simulink model "MPCRLTestPredict"  (R2023a)
settings: Solver=ode1  StartTime=0.0  StopTime=10  FixedStep=0.005  RelTol=1e-3  EnableMultiTasking=on
values from neighbouring files (symbols this model uses):
  bp = 5e-5*2    (= 0.0001)    [Copy_of_qube2_rotpen_param.m]    (also in MPCmodelinitial.m = 5e-05)
  br = 1e-3*2    (= 0.002)    [Copy_of_qube2_rotpen_param.m]    (also in MPCmodelinitial.m = 0.001)
  g = 9.81    [Copy_of_qube2_rotpen_param.m]    (also in MPCmodelinitial.m)
  Jp = mp*Lp^2/3    (= 0.0001464408)    [Copy_of_qube2_rotpen_param.m]    (also in MPCmodelinitial.m = 0.000133128)
  Jr = mr*r^2/3    (= 0.000251670833333)    [Copy_of_qube2_rotpen_param.m]    (also in MPCmodelinitial.m = 0.000228791666667)
  km = kt    (= 0.042)    [Copy_of_qube2_rotpen_param.m]    (also in MPCmodelinitial.m)
  kt = 0.042    [Copy_of_qube2_rotpen_param.m]    (also in MPCmodelinitial.m)
  l = Lp/2    (= 0.0645)    [Copy_of_qube2_rotpen_param.m]    (also in MPCmodelinitial.m)
  mp = 0.024*1.1    (= 0.0264)    [Copy_of_qube2_rotpen_param.m]    (also in MPCmodelinitial.m = 0.024)
  r = 0.085    [Copy_of_qube2_rotpen_param.m]    (also in MPCmodelinitial.m)
  Rm = 9.7    [Copy_of_qube2_rotpen_param.m]    (also in MPCmodelinitial.m = 8.4)
undefined symbols (not defined in the file or in its folder): ic_alpha0
libraries: simulink x6, rllib x3, sdolib x3, mpclib x2
settings Model: PacingRate=1000  ExtModeTrigDuration=10000  Creator=XIJ62  LastModifiedBy=lying
settings SolverCC: AlgebraicLoopSolver=TrustRegion  PositivePriorityOrder=on
settings DataIOCC: ReturnWorkspaceOutputs=off
settings DebuggingCC: UnconnectedInputMsg=warning  UnconnectedOutputMsg=warning  UnconnectedLineMsg=warning  ArithmeticOperatorsInVariantConditions=warning
settings ModelReferenceCC: EnableRefExpFcnMdlSchedulingChecks=on
settings SFSimCC: SimUseLocalCustomCode=off  CustomCodeUndefinedFunction=UseInterfaceOnly
settings RTWCC: Description=QUARC Win64 Target Using Toolchain  SystemTargetFile=quarc_win64.tlc  TemplateMakefile=quarc_default_tmf  RTWUseLocalCustomCode=off  Toolchain=QUARC win64 | nmake (64-bit Windows)  BuildConfiguration=Faster Runs  DLArmComputeVersion=19.05
settings CodeAppCC: StateflowObjectComments=on
settings STFCustomTargetCC: SystemTargetFile=quarc_win64.tlc
settings GRTTargetCC: ParMdlRefBuildCompliant=off  CompOptLevelCompliant=off  CombineOutputUpdateFcns=off  MatFileLogging=off  CPPClassGenCompliant=off  GRTInterface=on  ExtMode=on  ExtModeMexFile=quarc_comm
settings ConfigComp: CovMetricSettings=dswe

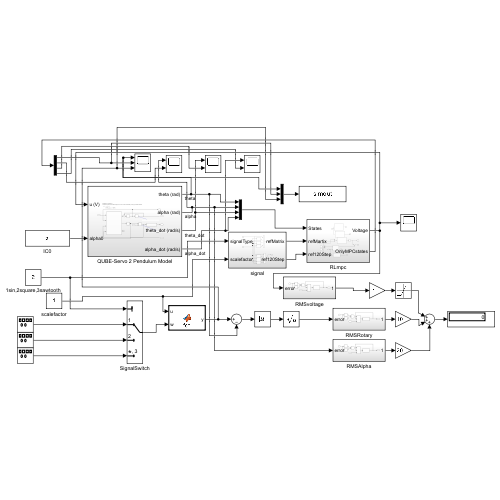
[thumbnail: Simulink's stored preview of the top-level diagram]
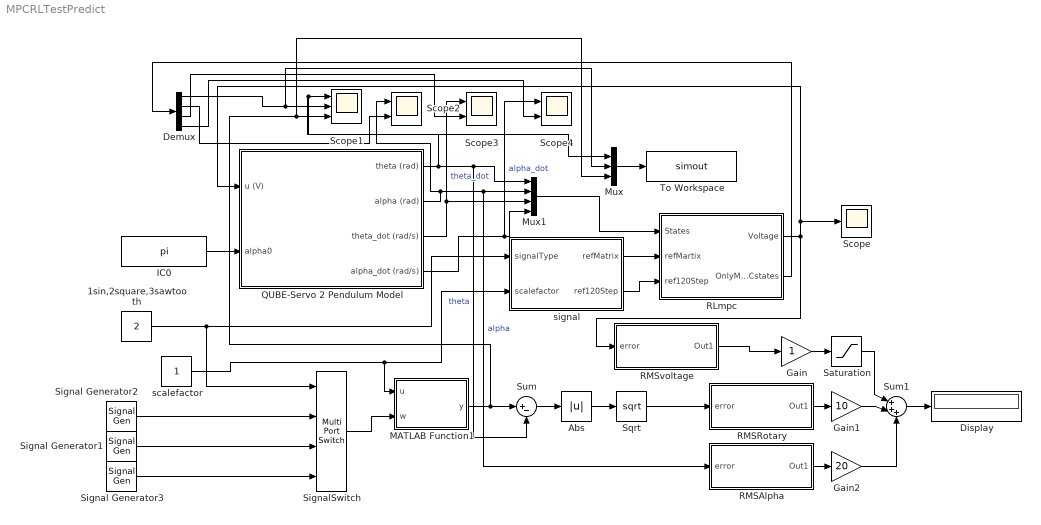
== system MPCRLTestPredict ==
  1sin,2square,3sawtooth : Constant  Value=2
  Abs : Abs  SaturateOnIntegerOverflow=off
  Demux : Demux
  Display : Display
  Gain : Gain
  Gain1 : Gain  Gain=10
  Gain2 : Gain  Gain=20
  IC0 : Constant  Value=pi
  MATLAB Function1 : MATLAB Function  TreatAsAtomicUnit=on
  Mux : Mux  Inputs=3
  Mux1 : Mux
  QUBE-Servo 2 Pendulum Model : Subsystem
  RLmpc : Subsystem
  RMSAlpha : Subsystem
  RMSRotary : Subsystem
  RMSvoltage : Subsystem
  Saturation : Saturate  UpperLimit=0  LowerLimit=0
  Scope : Scope
  Scope1 : Scope  NumInputPorts=3
  Scope2 : Scope  NumInputPorts=2
  Scope3 : Scope  NumInputPorts=2
  Scope4 : Scope  NumInputPorts=2
  Signal Generator1 : SignalGenerator  WaveForm=square  Amplitude=0.5  Units=rad/sec
  Signal Generator2 : SignalGenerator  Units=rad/sec
  Signal Generator3 : SignalGenerator  WaveForm=sawtooth  Units=rad/sec
  SignalSwitch : MultiPortSwitch  SaturateOnIntegerOverflow=off  InputSameDT=off
  Sqrt : Sqrt
  Sum : Sum  Inputs=|+-
  Sum1 : Sum  Inputs=|+++
  To Workspace : ToWorkspace  VariableName=simout  SaveFormat=Timeseries  SampleTime=-1
  scalefactor : Constant
  signal : Subsystem
  wires:
  RLmpc/1(Voltage) -> QUBE-Servo 2 Pendulum Model/1(u (V)), Scope/1, RMSvoltage/1(error)
  QUBE-Servo 2 Pendulum Model/1(theta (rad)) -> Mux/1, Scope1/1, Mux1/1, Sum/2  "theta"
  QUBE-Servo 2 Pendulum Model/2(alpha (rad)) -> Scope2/1, RMSAlpha/1(error), Mux1/2  "alpha"
  QUBE-Servo 2 Pendulum Model/3(theta_dot (rad/s)) -> Scope3/1, Mux1/3  "theta_dot"
  QUBE-Servo 2 Pendulum Model/4(alpha_dot (rad/s)) -> Scope4/1, Mux1/4  "alpha_dot"
  Mux1/1 -> RLmpc/1(States)
  IC0/1 -> QUBE-Servo 2 Pendulum Model/2(alpha0)
  RMSRotary/1(Out1) -> Gain1/1
  Sum/1 -> Abs/1
  scalefactor/1 -> MATLAB Function1/1(u), signal/2(scalefactor)
  signal/1(refMatrix) -> RLmpc/2(refMartix)
  signal/2(ref120Step) -> RLmpc/3(ref120Step)
  SignalSwitch/1 -> MATLAB Function1/2(w)
  MATLAB Function1/1(y) -> Sum/1, Mux/3, Scope1/3
  Signal Generator1/1 -> SignalSwitch/3
  Signal Generator2/1 -> SignalSwitch/2
  1sin,2square,3sawtooth/1 -> SignalSwitch/1, signal/1(signalType)
  RMSvoltage/1(Out1) -> Gain/1
  Signal Generator3/1 -> SignalSwitch/4
  RLmpc/2(OnlyMPCstates) -> Demux/1
  Demux/1 -> Mux/2, Scope1/2
  Demux/2 -> Scope2/2
  Demux/3 -> Scope3/2
  Demux/4 -> Scope4/2
  Mux/1 -> To Workspace/1
  RMSAlpha/1(Out1) -> Gain2/1
  Gain/1 -> Saturation/1
  Gain1/1 -> Sum1/2
  Gain2/1 -> Sum1/3
  Sum1/1 -> Display/1
  Abs/1 -> Sqrt/1
  Sqrt/1 -> RMSRotary/1(error)
  Saturation/1 -> Sum1/1

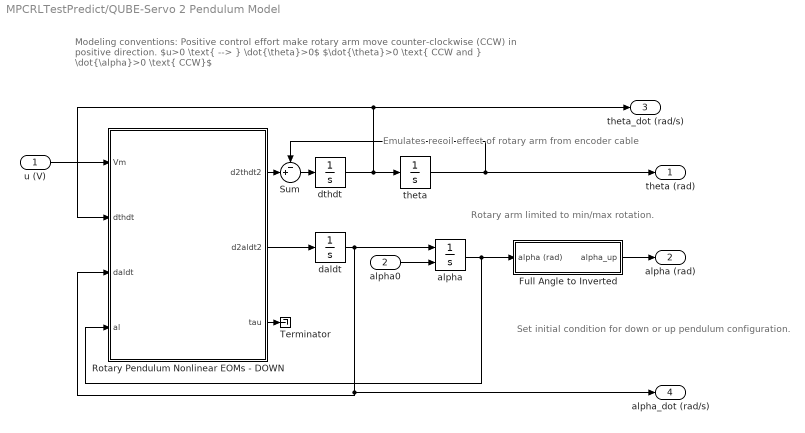
== system MPCRLTestPredict/QUBE-Servo 2 Pendulum Model ==
  note: Rotary arm limited to min/max rotation.
  note: Modeling conventions:
      | Positive control effort make rotary arm move counter-clockwise (CCW) in positive direction.
      | $u>0 \text{ --> } \dot{\theta}>0$
      | $\dot{\theta}>0 \text{ CCW and } \dot{\alpha}>0 \text{ CCW}$
  note: Set initial condition for down or up pendulum configuration.
  note: Emulates recoil effect of rotary arm from encoder cable
  u (V) : Inport
  alpha0 : Inport  Port=2
  Full Angle to Inverted : Subsystem
  Rotary Pendulum Nonlinear EOMs - DOWN : MATLAB Function  TreatAsAtomicUnit=on
  Sum : Sum  Inputs=-+|
  Terminator : Terminator
  alpha : Integrator  InitialConditionSource=external  InitialCondition=ic_alpha0
  daldt : Integrator
  dthdt : Integrator
  theta : Integrator  LimitOutput=on  UpperSaturationLimit=2  LowerSaturationLimit=-2
  theta (rad) : Outport  VectorParamsAs1DForOutWhenUnconnected=off
  alpha (rad) : Outport  Port=2  VectorParamsAs1DForOutWhenUnconnected=off
  theta_dot (rad/s) : Outport  Port=3  VectorParamsAs1DForOutWhenUnconnected=off
  alpha_dot (rad/s) : Outport  Port=4  VectorParamsAs1DForOutWhenUnconnected=off
  wires:
  daldt/1 -> Rotary Pendulum Nonlinear EOMs - DOWN/3(daldt), alpha_dot (rad/s)/1, alpha/1
  alpha/1 -> Full Angle to Inverted/1(alpha (rad)), Rotary Pendulum Nonlinear EOMs - DOWN/4(al)
  Rotary Pendulum Nonlinear EOMs - DOWN/2(d2aldt2) -> daldt/1
  dthdt/1 -> theta_dot (rad/s)/1, Rotary Pendulum Nonlinear EOMs - DOWN/2(dthdt), theta/1
  u (V)/1 -> Rotary Pendulum Nonlinear EOMs - DOWN/1(Vm)
  Rotary Pendulum Nonlinear EOMs - DOWN/3(tau) -> Terminator/1
  Full Angle to Inverted/1(alpha_up) -> alpha (rad)/1
  alpha0/1 -> alpha/2
  theta/1 -> theta (rad)/1, Sum/1
  Rotary Pendulum Nonlinear EOMs - DOWN/1(d2thdt2) -> Sum/2
  Sum/1 -> dthdt/1

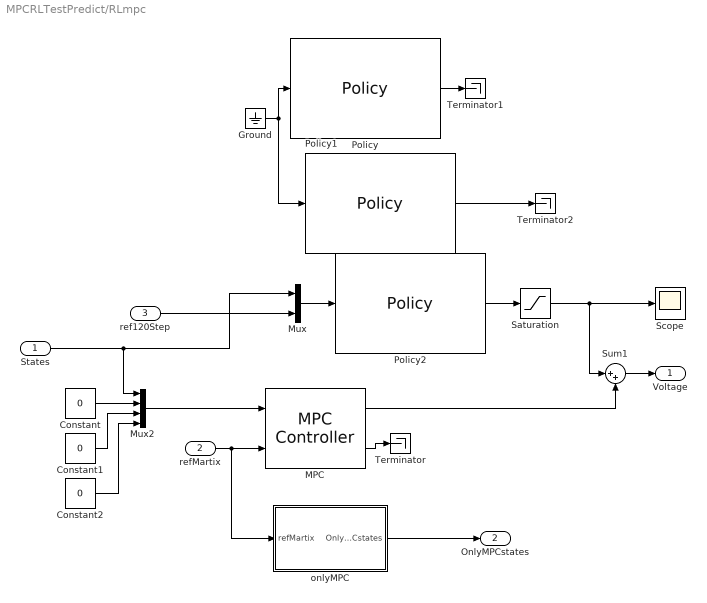
== system MPCRLTestPredict/RLmpc ==
  States : Inport
  refMartix : Inport  Port=2
  ref120Step : Inport  Port=3
  Constant : Constant  Value=0
  Constant1 : Constant  Value=0
  Constant2 : Constant  Value=0
  Ground : Ground
  MPC : mpclib/MPC Controller  SCDEnableBlockLinearizationSpecification=on  mpcobj=mpc1  is_multiple=0  enable_value=0  return_u0=off  updateMPCinCallerWorkspace=on  md_inport=off  mv_inport=off  uref_inport=off  return_cost=off  return_mvseq=off  return_qpstatus=off  return_xseq=off  return_state=on  return_ovseq=off  state_inport=on  umin_inport=off  umax_inport=off  ymin_inport=off  ymax_inport=off  cc_inport=off  ywt_inport=off  uwt_inport=off  duwt_inport=off  rhoeps_inport=off  pm_inport=off  MaximumP=10  HorizonChoice=FixedHorizon  n_ts=0.005  n_p=120  n_mv=1  n_md=0  n_ud=0  n_mo=4  n_uo=0  BlockDataType=double  SampleTimeInherited=off  switch_inport=off
  Mux : Mux  Inputs=2
  Mux2 : Mux
  Policy : rllib/Policy  MATFile=blockAgentData1.mat  SimUsingCodegen=off
  Policy1 : rllib/Policy  MATFile=blockAgentData2.mat  SimUsingCodegen=off
  Policy2 : rllib/Policy  MATFile=blockAgentData6.mat  SimUsingCodegen=off
  Saturation : Saturate  UpperLimit=10  LowerLimit=-10
  Scope : Scope
  Sum1 : Sum  Inputs=|++
  Terminator : Terminator
  Terminator1 : Terminator
  Terminator2 : Terminator
  onlyMPC : Subsystem
  Voltage : Outport
  OnlyMPCstates : Outport  Port=2
  wires:
  States/1 -> Mux2/1, Mux/1
  refMartix/1 -> onlyMPC/1(refMartix), MPC/2
  ref120Step/1 -> Mux/2
  MPC/2 -> Terminator/1
  MPC/1 -> Sum1/2
  Sum1/1 -> Voltage/1
  Constant1/1 -> Mux2/3
  Constant2/1 -> Mux2/4
  Constant/1 -> Mux2/2
  Mux2/1 -> MPC/1
  Saturation/1 -> Scope/1, Sum1/1
  onlyMPC/1(OnlyMPCstates) -> OnlyMPCstates/1
  Ground/1 -> Policy/1, Policy1/1
  Policy/1 -> Terminator1/1
  Policy1/1 -> Terminator2/1
  Mux/1 -> Policy2/1
  Policy2/1 -> Saturation/1

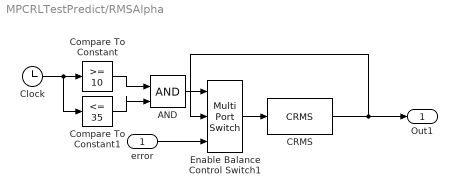
== system MPCRLTestPredict/RMSAlpha ==
  error : Inport
  AND : Logic  IconShape=distinctive  AllPortsSameDT=off  OutDataTypeStr=boolean
  CRMS : sdolib/RMS Blocks/CRMS
  Clock : Clock
  Compare To Constant : simulink/Logic and Bit Operations/Compare To Constant  relop=>=  const=10  OutDataTypeStr=boolean
  Compare To Constant1 : simulink/Logic and Bit Operations/Compare To Constant  relop=<=  const=35  OutDataTypeStr=boolean
  Enable Balance Control Switch1 : MultiPortSwitch  DataPortOrder=Zero-based contiguous  Inputs=2  zeroidx=on  SaturateOnIntegerOverflow=off  InputSameDT=off
  Out1 : Outport
  wires:
  Clock/1 -> Compare To Constant/1, Compare To Constant1/1
  Compare To Constant1/1 -> AND/2
  Compare To Constant/1 -> AND/1
  AND/1 -> Enable Balance Control Switch1/1
  Enable Balance Control Switch1/1 -> CRMS/1
  CRMS/1 -> Enable Balance Control Switch1/2, Out1/1
  error/1 -> Enable Balance Control Switch1/3

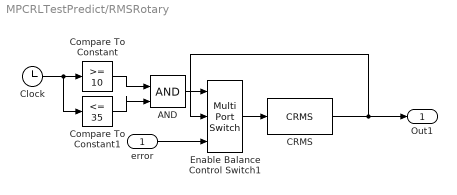
== system MPCRLTestPredict/RMSRotary ==
  error : Inport
  AND : Logic  IconShape=distinctive  AllPortsSameDT=off  OutDataTypeStr=boolean
  CRMS : sdolib/RMS Blocks/CRMS
  Clock : Clock
  Compare To Constant : simulink/Logic and Bit Operations/Compare To Constant  relop=>=  const=10  OutDataTypeStr=boolean
  Compare To Constant1 : simulink/Logic and Bit Operations/Compare To Constant  relop=<=  const=35  OutDataTypeStr=boolean
  Enable Balance Control Switch1 : MultiPortSwitch  DataPortOrder=Zero-based contiguous  Inputs=2  zeroidx=on  SaturateOnIntegerOverflow=off  InputSameDT=off
  Out1 : Outport
  wires:
  Clock/1 -> Compare To Constant/1, Compare To Constant1/1
  Compare To Constant1/1 -> AND/2
  Compare To Constant/1 -> AND/1
  AND/1 -> Enable Balance Control Switch1/1
  Enable Balance Control Switch1/1 -> CRMS/1
  CRMS/1 -> Enable Balance Control Switch1/2, Out1/1
  error/1 -> Enable Balance Control Switch1/3

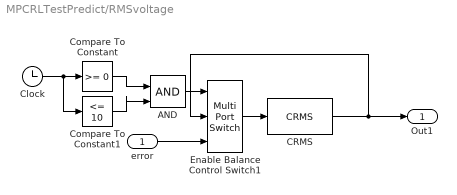
== system MPCRLTestPredict/RMSvoltage ==
  error : Inport
  AND : Logic  IconShape=distinctive  AllPortsSameDT=off  OutDataTypeStr=boolean
  CRMS : sdolib/RMS Blocks/CRMS
  Clock : Clock
  Compare To Constant : simulink/Logic and Bit Operations/Compare To Constant  relop=>=  const=0  OutDataTypeStr=boolean
  Compare To Constant1 : simulink/Logic and Bit Operations/Compare To Constant  relop=<=  const=10  OutDataTypeStr=boolean
  Enable Balance Control Switch1 : MultiPortSwitch  DataPortOrder=Zero-based contiguous  Inputs=2  zeroidx=on  SaturateOnIntegerOverflow=off  InputSameDT=off
  Out1 : Outport
  wires:
  Clock/1 -> Compare To Constant/1, Compare To Constant1/1
  Compare To Constant1/1 -> AND/2
  Compare To Constant/1 -> AND/1
  AND/1 -> Enable Balance Control Switch1/1
  Enable Balance Control Switch1/1 -> CRMS/1
  CRMS/1 -> Enable Balance Control Switch1/2, Out1/1
  error/1 -> Enable Balance Control Switch1/3

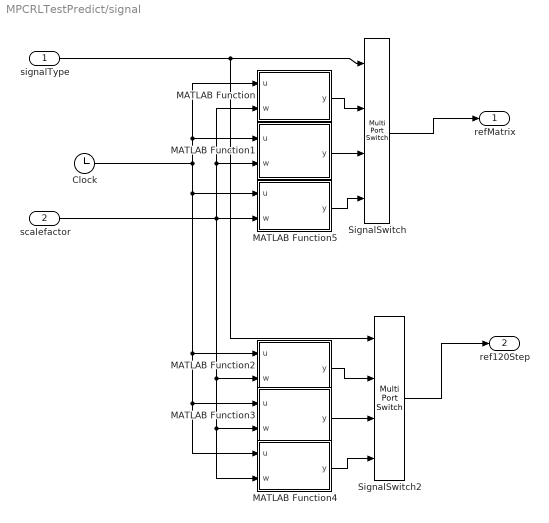
== system MPCRLTestPredict/signal ==
  signalType : Inport
  scalefactor : Inport  Port=2
  Clock : Clock
  MATLAB Function : MATLAB Function  TreatAsAtomicUnit=on
  MATLAB Function1 : MATLAB Function  TreatAsAtomicUnit=on
  MATLAB Function2 : MATLAB Function  TreatAsAtomicUnit=on
  MATLAB Function3 : MATLAB Function  TreatAsAtomicUnit=on
  MATLAB Function4 : MATLAB Function  TreatAsAtomicUnit=on
  MATLAB Function5 : MATLAB Function  TreatAsAtomicUnit=on
  SignalSwitch : MultiPortSwitch  SaturateOnIntegerOverflow=off  InputSameDT=off
  SignalSwitch2 : MultiPortSwitch  SaturateOnIntegerOverflow=off  InputSameDT=off
  refMatrix : Outport
  ref120Step : Outport  Port=2
  wires:
  signalType/1 -> SignalSwitch2/1, SignalSwitch/1
  MATLAB Function/1(y) -> SignalSwitch/2
  scalefactor/1 -> MATLAB Function/2(w), MATLAB Function1/2(w), MATLAB Function3/2(w), MATLAB Function4/2(w), MATLAB Function2/2(w), MATLAB Function5/2(w)
  MATLAB Function2/1(y) -> SignalSwitch2/2
  MATLAB Function1/1(y) -> SignalSwitch/3
  SignalSwitch/1 -> refMatrix/1
  SignalSwitch2/1 -> ref120Step/1
  MATLAB Function3/1(y) -> SignalSwitch2/3
  MATLAB Function4/1(y) -> SignalSwitch2/4
  Clock/1 -> MATLAB Function/1(u), MATLAB Function1/1(u), MATLAB Function5/1(u), MATLAB Function4/1(u), MATLAB Function3/1(u), MATLAB Function2/1(u)
  MATLAB Function5/1(y) -> SignalSwitch/4

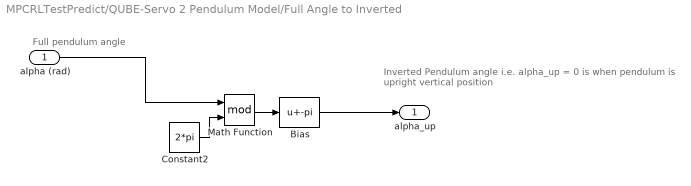
== system MPCRLTestPredict/QUBE-Servo 2 Pendulum Model/Full Angle to Inverted ==
  note: Inverted Pendulum angle
      | i.e. alpha_up = 0 is when pendulum is upright vertical position
  note: Full pendulum angle
  alpha (rad) : Inport
  Bias : Bias  Bias=-pi  SaturateOnIntegerOverflow=off
  Constant2 : Constant  Value=2*pi
  Math Function : Math  Operator=mod  SignedPower=on
  alpha_up : Outport  VectorParamsAs1DForOutWhenUnconnected=off
  wires:
  Constant2/1 -> Math Function/2
  Bias/1 -> alpha_up/1
  alpha (rad)/1 -> Math Function/1
  Math Function/1 -> Bias/1

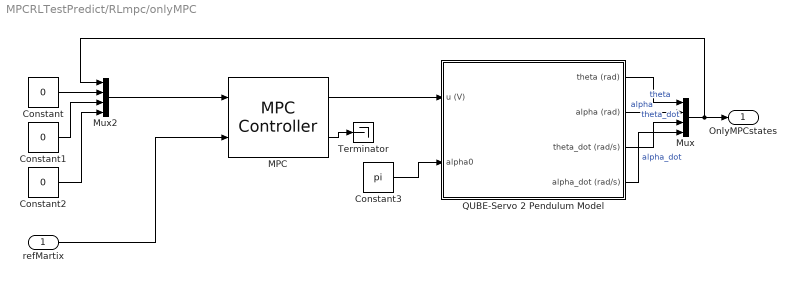
== system MPCRLTestPredict/RLmpc/onlyMPC ==
  refMartix : Inport
  Constant : Constant  Value=0
  Constant1 : Constant  Value=0
  Constant2 : Constant  Value=0
  Constant3 : Constant  Value=pi
  MPC : mpclib/MPC Controller  SCDEnableBlockLinearizationSpecification=on  mpcobj=mpc1  is_multiple=0  enable_value=0  return_u0=off  updateMPCinCallerWorkspace=on  md_inport=off  mv_inport=off  uref_inport=off  return_cost=off  return_mvseq=off  return_qpstatus=off  return_xseq=off  return_state=on  return_ovseq=off  state_inport=on  umin_inport=off  umax_inport=off  ymin_inport=off  ymax_inport=off  cc_inport=off  ywt_inport=off  uwt_inport=off  duwt_inport=off  rhoeps_inport=off  pm_inport=off  MaximumP=10  HorizonChoice=FixedHorizon  n_ts=0.005  n_p=120  n_mv=1  n_md=0  n_ud=0  n_mo=4  n_uo=0  BlockDataType=double  SampleTimeInherited=off  switch_inport=off
  Mux : Mux
  Mux2 : Mux
  QUBE-Servo 2 Pendulum Model : Subsystem
  Terminator : Terminator
  OnlyMPCstates : Outport
  wires:
  MPC/2 -> Terminator/1
  Constant/1 -> Mux2/2
  refMartix/1 -> MPC/2
  Mux/1 -> Mux2/1, OnlyMPCstates/1
  Constant2/1 -> Mux2/4
  Mux2/1 -> MPC/1
  Constant1/1 -> Mux2/3
  MPC/1 -> QUBE-Servo 2 Pendulum Model/1(u (V))
  Constant3/1 -> QUBE-Servo 2 Pendulum Model/2(alpha0)
  QUBE-Servo 2 Pendulum Model/1(theta (rad)) -> Mux/1  "theta"
  QUBE-Servo 2 Pendulum Model/2(alpha (rad)) -> Mux/2  "alpha"
  QUBE-Servo 2 Pendulum Model/3(theta_dot (rad/s)) -> Mux/3  "theta_dot"
  QUBE-Servo 2 Pendulum Model/4(alpha_dot (rad/s)) -> Mux/4  "alpha_dot"

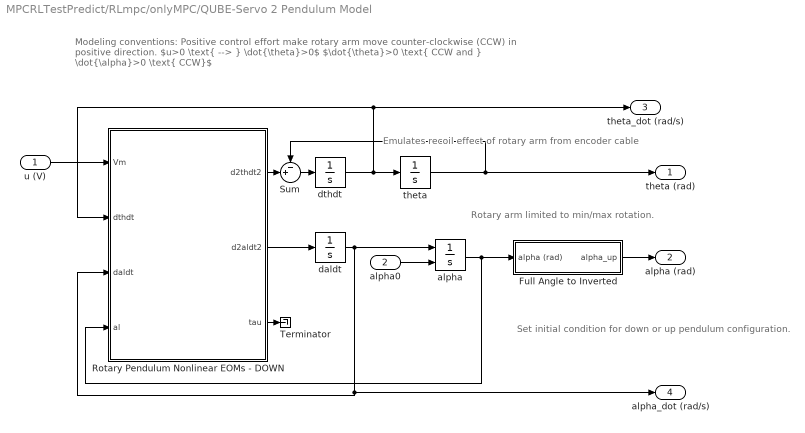
== system MPCRLTestPredict/RLmpc/onlyMPC/QUBE-Servo 2 Pendulum Model ==
  note: Rotary arm limited to min/max rotation.
  note: Modeling conventions:
      | Positive control effort make rotary arm move counter-clockwise (CCW) in positive direction.
      | $u>0 \text{ --> } \dot{\theta}>0$
      | $\dot{\theta}>0 \text{ CCW and } \dot{\alpha}>0 \text{ CCW}$
  note: Set initial condition for down or up pendulum configuration.
  note: Emulates recoil effect of rotary arm from encoder cable
  u (V) : Inport
  alpha0 : Inport  Port=2
  Full Angle to Inverted : Subsystem
  Rotary Pendulum Nonlinear EOMs - DOWN : MATLAB Function  TreatAsAtomicUnit=on
  Sum : Sum  Inputs=-+|
  Terminator : Terminator
  alpha : Integrator  InitialConditionSource=external  InitialCondition=ic_alpha0
  daldt : Integrator
  dthdt : Integrator
  theta : Integrator  LimitOutput=on  UpperSaturationLimit=2  LowerSaturationLimit=-2
  theta (rad) : Outport  VectorParamsAs1DForOutWhenUnconnected=off
  alpha (rad) : Outport  Port=2  VectorParamsAs1DForOutWhenUnconnected=off
  theta_dot (rad/s) : Outport  Port=3  VectorParamsAs1DForOutWhenUnconnected=off
  alpha_dot (rad/s) : Outport  Port=4  VectorParamsAs1DForOutWhenUnconnected=off
  wires:
  daldt/1 -> Rotary Pendulum Nonlinear EOMs - DOWN/3(daldt), alpha_dot (rad/s)/1, alpha/1
  alpha/1 -> Full Angle to Inverted/1(alpha (rad)), Rotary Pendulum Nonlinear EOMs - DOWN/4(al)
  Rotary Pendulum Nonlinear EOMs - DOWN/2(d2aldt2) -> daldt/1
  dthdt/1 -> theta_dot (rad/s)/1, Rotary Pendulum Nonlinear EOMs - DOWN/2(dthdt), theta/1
  u (V)/1 -> Rotary Pendulum Nonlinear EOMs - DOWN/1(Vm)
  Rotary Pendulum Nonlinear EOMs - DOWN/3(tau) -> Terminator/1
  Full Angle to Inverted/1(alpha_up) -> alpha (rad)/1
  alpha0/1 -> alpha/2
  theta/1 -> theta (rad)/1, Sum/1
  Rotary Pendulum Nonlinear EOMs - DOWN/1(d2thdt2) -> Sum/2
  Sum/1 -> dthdt/1

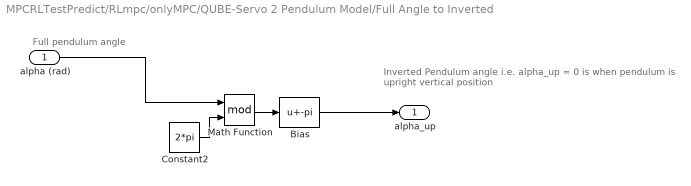
== system MPCRLTestPredict/RLmpc/onlyMPC/QUBE-Servo 2 Pendulum Model/Full Angle to Inverted ==
  note: Inverted Pendulum angle
      | i.e. alpha_up = 0 is when pendulum is upright vertical position
  note: Full pendulum angle
  alpha (rad) : Inport
  Bias : Bias  Bias=-pi  SaturateOnIntegerOverflow=off
  Constant2 : Constant  Value=2*pi
  Math Function : Math  Operator=mod  SignedPower=on
  alpha_up : Outport  VectorParamsAs1DForOutWhenUnconnected=off
  wires:
  Constant2/1 -> Math Function/2
  Bias/1 -> alpha_up/1
  alpha (rad)/1 -> Math Function/1
  Math Function/1 -> Bias/1

== matlab function MPCRLTestPredict/signal/MATLAB Function2 ==
  data: u input; y output; w input
function y = SignalPredictRLSin(u,w)
    Np=120; %Prediction horizon
    Signal=zeros(120,1);
    t=u;
    for (k=1:120)
        Signal(k)=sin(t+0.005*k-0.005);
    end
    y = Signal*w;
end

== matlab function MPCRLTestPredict/signal/MATLAB Function1 ==
  data: u input; y output; w input
function y = SignalMatrixSquare(u,w)
    Signal=zeros(120,4);
    for (k=1:120)
        t=floor((u+0.005*k-0.005)/pi);
        Signal(k,1)=mod(t,2)-0.5;
    end
    y = Signal*w;
end

== matlab function MPCRLTestPredict/signal/MATLAB Function3 ==
  data: u input; y output; w input
function y = SignalPredictSquare(u,w)
    Signal=zeros(120,1);
    for (k=1:120)
        t=floor((u+0.005*k-0.005)/pi);
        Signal(k)=mod(t,2)-0.5;
    end
    y = Signal*w;
end

== matlab function MPCRLTestPredict/MATLAB Function1 ==
  data: u input; y output; w input
function y = fcn(u,w)

y = u*w;

== matlab function MPCRLTestPredict/signal/MATLAB Function4 ==
  data: u input; y output; w input
function y = SignalPredictSawtooth(u,w)
    Signal=zeros(120,1);
    for (k=1:120)
        Signal(k)=1-1/pi*mod((u+0.005*k-0.005),2*pi);
    end
    y = Signal*w;
end

== matlab function MPCRLTestPredict/signal/MATLAB Function5 ==
  data: u input; y output; w input
function y = SignalMatrixSawtooth(u,w)
    Signal=zeros(120,4);
    for (k=1:120)
        Signal(k,1)=1-1/pi*mod((u+0.005*k-0.005),2*pi);
    end
    y = Signal*w;
end

== matlab function MPCRLTestPredict/RLmpc/onlyMPC/QUBE-Servo 2 Pendulum Model/Rotary Pendulum Nonlinear EOMs - DOWN ==
  data: Vm input size=1; d2thdt2 output size=1; d2aldt2 output size=1; dthdt input size=1; daldt input size=1; Jp parameter; Jr parameter; l parameter; mp parameter; br parameter; bp parameter; r parameter; kt parameter; km parameter; Rm parameter; al input size=1; g parameter; tau output
function [d2thdt2,d2aldt2,tau] = pen_nonlin_eoms(Vm, dthdt, daldt, Jp, Jr, l, mp, br, bp, r, kt, km, Rm, al, g)

% Convert voltage to torque input
tau = (Vm - km*dthdt)/Rm;
tau=kt*tau;
% Denominator
Jt = Jr*Jp + Jp^2*sin(al)^2 - mp^2*r^2*l^2*cos(al)^2;
% Nonlinear equations of motion for generic rotary pendulum (i.e. furuta)
% Terms from EOM solving
term1 = tau - br*dthdt + 2*Jp*sin(al)*cos(al)*dthdt*daldt + mp*r*l*sin(al)*daldt^2;
term2 = -bp*daldt - Jp*sin(al)*cos(al)*daldt^2 - mp*g*l*sin(al);
% Torque to rotary arm position)
d2thdt2 = 1/Jt*( Jp*term1 - mp*r*l*cos(al)*term2);
% Torque to pendulum angle position
d2aldt2 = 1/Jt*(-mp*r*l*cos(al)*term1 + (Jr+Jp*sin(al)^2)*term2);

== matlab function MPCRLTestPredict/QUBE-Servo 2 Pendulum Model/Rotary Pendulum Nonlinear EOMs - DOWN ==
  data: Vm input size=1; d2thdt2 output size=1; d2aldt2 output size=1; dthdt input size=1; daldt input size=1; Jp parameter; Jr parameter; l parameter; mp parameter; br parameter; bp parameter; r parameter; kt parameter; km parameter; Rm parameter; al input size=1; g parameter; tau output
function [d2thdt2,d2aldt2,tau] = pen_nonlin_eoms(Vm, dthdt, daldt, Jp, Jr, l, mp, br, bp, r, kt, km, Rm, al, g)

% Convert voltage to torque input
tau = (Vm - km*dthdt)/Rm;
tau=kt*tau;
% Denominator
Jt = Jr*Jp + Jp^2*sin(al)^2 - mp^2*r^2*l^2*cos(al)^2;
% Nonlinear equations of motion for generic rotary pendulum (i.e. furuta)
% Terms from EOM solving
term1 = tau - br*dthdt + 2*Jp*sin(al)*cos(al)*dthdt*daldt + mp*r*l*sin(al)*daldt^2;
term2 = -bp*daldt - Jp*sin(al)*cos(al)*daldt^2 - mp*g*l*sin(al);
% Torque to rotary arm position)
d2thdt2 = 1/Jt*( Jp*term1 - mp*r*l*cos(al)*term2);
% Torque to pendulum angle position
d2aldt2 = 1/Jt*(-mp*r*l*cos(al)*term1 + (Jr+Jp*sin(al)^2)*term2);

== matlab function MPCRLTestPredict/signal/MATLAB Function ==
  data: u input; y output; w input
function y = SignalMatrixSin(u,w)
    Np=120; %Prediction horizon
    Signal=zeros(120,4);
    t=u;
    for (k=1:120)
        Signal(k,1)=sin(t+0.005*k-0.005);
    end
    y = Signal*w;
end
